simulink model "motor1"  (R2023a)
settings: Solver=VariableStepAuto  StartTime=0.0  StopTime=10.0  RelTol=1e-3
settings Model: Creator=mrrom  LastModifiedBy=mrrom

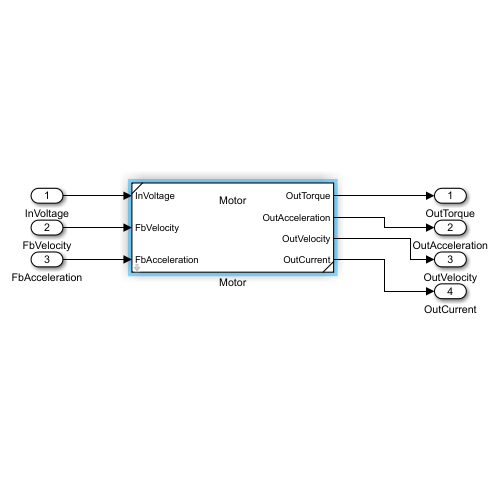
[thumbnail: Simulink's stored preview of the top-level diagram]
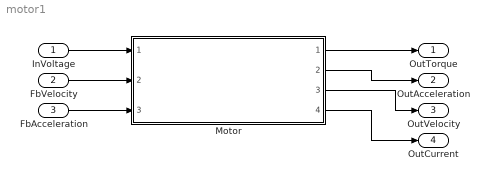
== system motor1 ==
  InVoltage : Inport
  FbVelocity : Inport  Port=2
  FbAcceleration : Inport  Port=3
  Motor : Subsystem  ReferencedSubsystem=Motor  kw=62.8  km=16e-3  motor_nominal_voltage=24  vis_friction_coef_motor=0.0025
  OutTorque : Outport
  OutAcceleration : Outport  Port=2
  OutVelocity : Outport  Port=3
  OutCurrent : Outport  Port=4
  wires:
  InVoltage/1 -> Motor/1
  FbVelocity/1 -> Motor/2
  FbAcceleration/1 -> Motor/3
  Motor/1 -> OutTorque/1
  Motor/2 -> OutAcceleration/1
  Motor/3 -> OutVelocity/1
  Motor/4 -> OutCurrent/1
